simulink model "simulation"  (R2019b)
settings: Solver=VariableStepAuto  StartTime=0.0  StopTime=400  RelTol=1e-3
values from neighbouring files (symbols this model uses):
  Kc = 1    [cw_6.m]
  Ki = 0.2    [cw_6.m]
  Kp = 2    [cw_6.m]
  u_sat = 10    [cw_6.m]
  y_ref = 10    [cw_6.m]
settings Model: Creator=kacpe  LastModifiedBy=kacpe

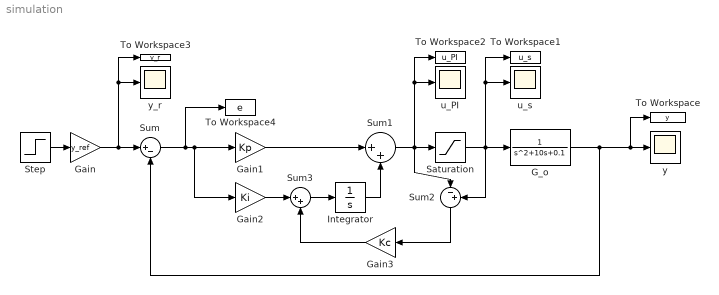
== system simulation ==
  G_o : TransferFcn  Denominator=[1 10 0.1]
  Gain : Gain  Gain=y_ref
  Gain1 : Gain  Gain=Kp
  Gain2 : Gain  Gain=Ki
  Gain3 : Gain  Gain=Kc
  Integrator : Integrator
  Saturation : Saturate  UpperLimit=u_sat  LowerLimit=-u_sat
  Step : Step  SampleTime=0
  Sum : Sum  Inputs=|+-
  Sum1 : Sum  Inputs=|++
  Sum2 : Sum  Inputs=|-+
  Sum3 : Sum  Inputs=|++
  To Workspace : ToWorkspace  VariableName=y  SampleTime=-1
  To Workspace1 : ToWorkspace  VariableName=u_s  SampleTime=-1
  To Workspace2 : ToWorkspace  VariableName=u_PI  SampleTime=-1
  To Workspace3 : ToWorkspace  VariableName=y_r  SampleTime=-1
  To Workspace4 : ToWorkspace  VariableName=e  SampleTime=-1
  u_PI : Scope
  "u_s " : Scope
  "y " : Scope
  y_r : Scope
  wires:
  Gain/1 -> To Workspace3/1, y_r/1, Sum/1
  Sum/1 -> To Workspace4/1, Gain2/1, Gain1/1
  Sum1/1 -> Sum2/1, Saturation/1, u_PI/1, To Workspace2/1
  Saturation/1 -> Sum2/2, To Workspace1/1, "u_s "/1, G_o/1
  G_o/1 -> To Workspace/1, "y "/1, Sum/2
  Step/1 -> Gain/1
  Integrator/1 -> Sum1/2
  Gain1/1 -> Sum1/1
  Sum2/1 -> Gain3/1
  Gain2/1 -> Sum3/1
  Sum3/1 -> Integrator/1
  Gain3/1 -> Sum3/2
